simulink model "engineModelF16TestHarness"  (R2024a)
settings: configuration reference "standardSILConfiguraitonParams" (kept outside this file)
libraries: aerolibatmos2 x1
settings Model: Creator=jerem  LastModifiedBy=jerem
settings ConfigSetRef: SourceName=standardSILConfiguraitonParams  SourceLocation=Base Workspace

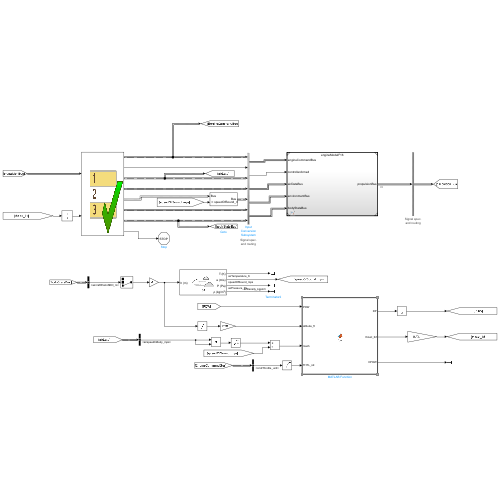
[thumbnail: Simulink's stored preview of the top-level diagram]
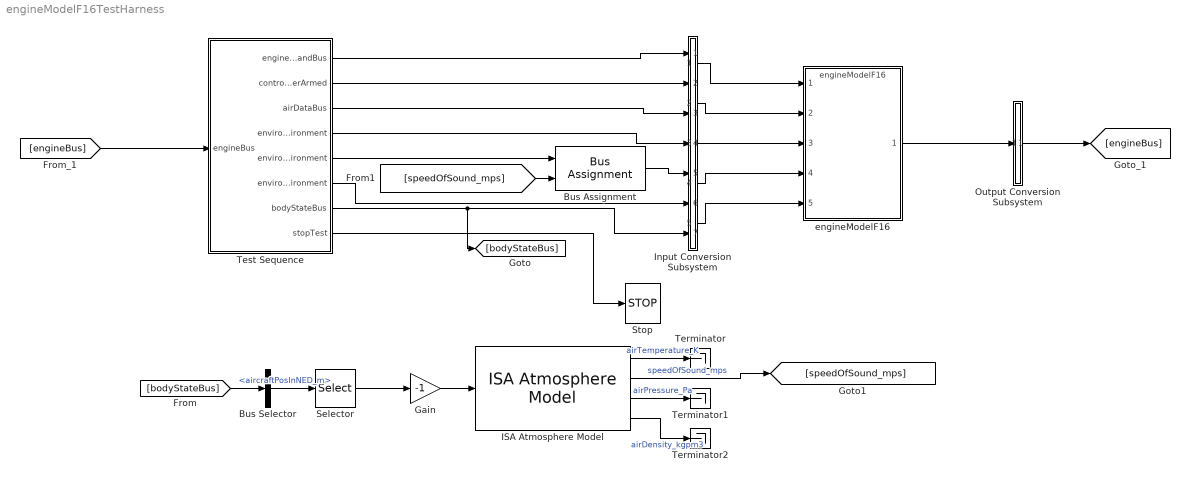
== system engineModelF16TestHarness ==
  Bus Assignment : BusAssignment  AssignedSignals=speedOfSound_mps
  Bus Selector : BusSelector  OutputSignals=aircraftPosInNED_m
  Gain : Gain  Gain=-1
  ISA Atmosphere Model : aerolibatmos2/ISA Atmosphere Model  useExtended=off  action=Warning  custom=off  viscosityOut=off  g=9.80665  gamma=1.4  R=287.0531  L=0.0065  h_trop=11000  h_strat=20000  rho0=1.225  P0=101325  T0=288.15  h0=0  S=110.4  Tref=273.15  muref=1.716e-5
  Input Conversion Subsystem : Subsystem  Tag=__SLT_ICS__  Description=|
      | Signal spec.
      | and routing
      settings: AttributesFormatString=%<Description>
  Output Conversion Subsystem : Subsystem  Tag=__SLT_OCS__  Description=|
      | Signal spec.
      | and routing
      mask init:
      | ICDictionary = get_param(bdroot, 'DataDictionary');
      | if isempty(ICDictionary)
      |    ICScope = Simulink.data.BaseWorkspace;
      | else
      |    ICScope = Simulink.data.DataDictionary(ICDictionary);
      | end
      | 
      | IC1 = Simulink.Bus.createMATLABStruct('EngineBus', [], [1 1], ICScope);
      settings: AttributesFormatString=%<Description>
  Selector : Selector  InputPortWidth=3  IndexOptions=Index vector (dialog)  Indices=3  OutputSizes=1
  Stop : Stop
  Terminator : Terminator
  Terminator1 : Terminator
  Terminator2 : Terminator
  Test Sequence : Test Sequence  TreatAsAtomicUnit=on
  engineModelF16 : ModelReference  ModelNameDialog=engineModelF16  SimulationMode=Normal  ModelReferenceVersion=1.84
  wires:
  Test Sequence/1(engineCommandBus) -> Input Conversion Subsystem/1(Inport_1)
  Test Sequence/2(controllerArmed) -> Input Conversion Subsystem/2(Inport_2)
  Test Sequence/3(airDataBus) -> Input Conversion Subsystem/3(Inport_3)
  Test Sequence/4(environmentBus_EarthEnvironment) -> Input Conversion Subsystem/4(Inport_4)
  Test Sequence/6(environmentBus_TerrainEnvironment) -> Input Conversion Subsystem/6(Inport_6)
  Test Sequence/7(bodyStateBus) -> [bodyStateBus], Input Conversion Subsystem/7(Inport_7)
  [engineBus] -> Test Sequence/1(engineBus)
  Output Conversion Subsystem/1(Outport_1) -> [engineBus]
  Input Conversion Subsystem/1(Outport_1) -> engineModelF16/1
  Input Conversion Subsystem/2(Outport_2) -> engineModelF16/2
  Input Conversion Subsystem/3(Outport_3) -> engineModelF16/3
  Input Conversion Subsystem/4(Outport_4) -> engineModelF16/4
  Input Conversion Subsystem/5(Outport_5) -> engineModelF16/5
  engineModelF16/1 -> Output Conversion Subsystem/1(Inport_1)
  Test Sequence/8(stopTest) -> Stop/1
  [bodyStateBus] -> Bus Selector/1
  Bus Selector/1 -> Selector/1  "<aircraftPosInNED_m>"
  Selector/1 -> Gain/1
  Gain/1 -> ISA Atmosphere Model/1
  ISA Atmosphere Model/1 -> Terminator/1  "airTemperature_K"
  ISA Atmosphere Model/3 -> Terminator1/1  "airPressure_Pa"
  ISA Atmosphere Model/4 -> Terminator2/1  "airDensity_kgpm3"
  ISA Atmosphere Model/2 -> [speedOfSound_mps]  "speedOfSound_mps"
  Test Sequence/5(environmentBus_AirEnvironment) -> Bus Assignment/1
  [speedOfSound_mps] -> Bus Assignment/2
  Bus Assignment/1 -> Input Conversion Subsystem/5(Inport_5)

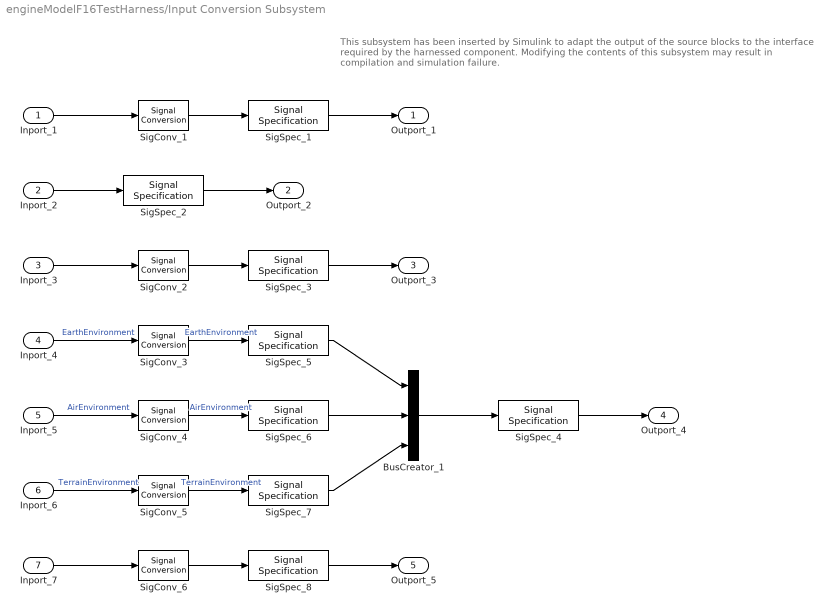
== system engineModelF16TestHarness/Input Conversion Subsystem ==
  note: This subsystem has been inserted by Simulink to adapt the output of the source blocks to the interface required by the harnessed component.
      |  Modifying the contents of this subsystem may result in compilation and simulation failure.
  Inport_1 : Inport
  Inport_2 : Inport  Port=2
  Inport_3 : Inport  Port=3
  Inport_4 : Inport  Port=4
  Inport_5 : Inport  Port=5
  Inport_6 : Inport  Port=6
  Inport_7 : Inport  Port=7
  BusCreator_1 : BusCreator  Inputs=3  OutDataTypeStr=Bus: EnvironmentBus
  SigConv_1 : SignalConversion  ConversionOutput=Virtual bus  OverrideOpt=off
  SigConv_2 : SignalConversion  ConversionOutput=Virtual bus  OverrideOpt=off
  SigConv_3 : SignalConversion  ConversionOutput=Nonvirtual bus  OverrideOpt=off
  SigConv_4 : SignalConversion  ConversionOutput=Nonvirtual bus  OverrideOpt=off
  SigConv_5 : SignalConversion  ConversionOutput=Nonvirtual bus  OverrideOpt=off
  SigConv_6 : SignalConversion  ConversionOutput=Virtual bus  OverrideOpt=off
  SigSpec_1 : SignalSpecification  OutDataTypeStr=Bus: EngineCommandBus  SampleTime=[-1, 0]
  SigSpec_2 : SignalSpecification  OutDataTypeStr=double  Dimensions=[1]  SampleTime=[-1, 0]
  SigSpec_3 : SignalSpecification  OutDataTypeStr=Bus: AirData  SampleTime=[-1, 0]
  SigSpec_4 : SignalSpecification  OutDataTypeStr=Bus: EnvironmentBus  SampleTime=[-1, 0]
  SigSpec_5 : SignalSpecification  OutDataTypeStr=Bus: EarthEnvironmentBus  Dimensions=[1]  SampleTime=[-1, 0]  BusOutputAsStruct=on
  SigSpec_6 : SignalSpecification  OutDataTypeStr=Bus: AirEnvironmentBus  Dimensions=[1]  SampleTime=[-1, 0]  BusOutputAsStruct=on
  SigSpec_7 : SignalSpecification  OutDataTypeStr=Bus: TerrainEnvironmentBus  Dimensions=[1]  SampleTime=[-1, 0]  BusOutputAsStruct=on
  SigSpec_8 : SignalSpecification  OutDataTypeStr=Bus: BodyStateBus  SampleTime=[-1, 0]
  Outport_1 : Outport
  Outport_2 : Outport  Port=2
  Outport_3 : Outport  Port=3
  Outport_4 : Outport  Port=4
  Outport_5 : Outport  Port=5
  wires:
  SigSpec_1/1 -> Outport_1/1
  SigConv_1/1 -> SigSpec_1/1
  Inport_1/1 -> SigConv_1/1
  SigSpec_2/1 -> Outport_2/1
  Inport_2/1 -> SigSpec_2/1
  SigSpec_3/1 -> Outport_3/1
  SigConv_2/1 -> SigSpec_3/1
  Inport_3/1 -> SigConv_2/1
  SigSpec_4/1 -> Outport_4/1
  BusCreator_1/1 -> SigSpec_4/1
  SigSpec_5/1 -> BusCreator_1/1
  SigConv_3/1 -> SigSpec_5/1  "EarthEnvironment"
  Inport_4/1 -> SigConv_3/1  "EarthEnvironment"
  SigSpec_6/1 -> BusCreator_1/2
  SigConv_4/1 -> SigSpec_6/1  "AirEnvironment"
  Inport_5/1 -> SigConv_4/1  "AirEnvironment"
  SigSpec_7/1 -> BusCreator_1/3
  SigConv_5/1 -> SigSpec_7/1  "TerrainEnvironment"
  Inport_6/1 -> SigConv_5/1  "TerrainEnvironment"
  SigSpec_8/1 -> Outport_5/1
  SigConv_6/1 -> SigSpec_8/1
  Inport_7/1 -> SigConv_6/1

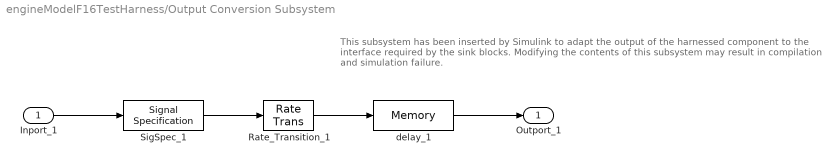
== system engineModelF16TestHarness/Output Conversion Subsystem ==
  note: This subsystem has been inserted by Simulink to adapt the output of the harnessed component to the interface required by the sink blocks.
      |  Modifying the contents of this subsystem may result in compilation and simulation failure.
  Inport_1 : Inport
  Rate_Transition_1 : RateTransition  OutPortSampleTimeOpt=Inherit
  SigSpec_1 : SignalSpecification  OutDataTypeStr=Bus: EngineBus  Dimensions=[1]
  delay_1 : Memory  InitialCondition=IC1
  Outport_1 : Outport
  wires:
  Inport_1/1 -> SigSpec_1/1
  SigSpec_1/1 -> Rate_Transition_1/1
  Rate_Transition_1/1 -> delay_1/1
  delay_1/1 -> Outport_1/1

== matlab function engineModelF16TestHarness/MATLAB Function ==
  data: POW input; DP output; altitude_ft input; mach input; thrust_lbf output; THTL_nd input; CPOW output
function [DP,thrust_lbf, CPOW] = fcn(POW, altitude_ft, mach, THTL_nd)

coder.extrinsic("PDOT")
coder.extrinsic("THRUST")
coder.extrinsic("TGEAR")
thrust_lbf = 0;
CPOW = 0;
DP = 0;

CPOW = TGEAR(THTL_nd);
thrust_lbf = THRUST(POW,altitude_ft, mach);
DP = PDOT(POW, CPOW);

== stateflow chart engineModelF16TestHarness/Test Sequence ==
  state Scenario_1
    state Initialize
      %% Initialize data outputs.
      engineCommandBus.cmdThrottle_unit = 0;
      controllerArmed = 0;
      airDataBus.airspeedInBody_mps = zeros(3,1);
      airDataBus.alpha_rad = 0;
      airDataBus.beta_rad = 0;
      environmentBus_EarthEnvironment.gravityScalar_mps2 = 0;
      environmentBus_EarthEnvironment.worldMagneticFieldInNED_nT = zeros(3,1);
      environmentBus_AirEnvironment.airTemperature_K = 0;
      environmentBus_AirEnvironment.airPressure_Pa = 0;
      environmentBus_AirEnvironment.airDensity_kgpm3 = 0;
      environmentBus_AirEnvironment.windSpeedInNED_mps = zeros(3,1);
      environmentBus_AirEnvironment.speedOfSound_mps = 0;
      environmentBus_AirEnvironment.windsAloftInNED_mps = zeros(3,1);
      environmentBus_AirEnvironment.gustInNED_mps = zeros(3,1);
      environmentBus_AirEnvironment.turbulenceInNED_mps = zeros(3,1);
      environmentBus_TerrainEnvironment.terrainHeightInNED_m = 0;
      bodyStateBus.aircraftVelInNED_mps = zeros(3,1);
      bodyStateBus.aircraftPosInNED_m = zeros(3,1);
      bodyStateBus.aircraftEulerAngles_rad = zeros(3,1);
      bodyStateBus.aircraftVelInBody_mps = zeros(3,1);
      bodyStateBus.aircraftAngVelInBody_radps = zeros(3,1);
      bodyStateBus.aircraftAngAccelInBody_radps2 = zeros(3,1);
      bodyStateBus.aircraftAccelInBody_mps2 = zeros(3,1);
      bodyStateBus.DCM_be = zeros(3,3);
      stopTest = false;
    state commandThrottle
      engineCommandBus.cmdThrottle_unit = 0.02;
    state verifyControllerDisarm
      verify(isClose(propulsionBus.engineForcesMoments.forcesInBody_N(1),0))
    state armController
      controllerArmed = 1;
      engineCommandBus.cmdThrottle_unit = 0.2;
    state verifyThorttle
      verify(isClose(thrust_lbf, propulsionBus.engineForcesMoments.forcesInBody_N(1), 'atol', 1))
    state maxCommandThrottle
      engineCommandBus.cmdThrottle_unit=10.5;
      settings: description=try out of range throttle > 1.0
    state verifyMaxThrust
      verify(propulsionBus.engineForcesMoments.forcesInBody_N(1) < 130000) % 130kN is what is listed on google as max thrust
      verify(isClose(thrust_lbf, propulsionBus.engineForcesMoments.forcesInBody_N(1), 'atol', 1))
      settings: description=max thrust taken from 5279e61a468c5ead544c0289877962cbf8e0459c
    state simulateAirspeed
      airDataBus.airspeedInBody_mps(1) = 100;
      bodyStateBus.aircraftPosInNED_m(3) = -1000;
    state verifyWithAirspeed
      verify(isClose(thrust_lbf, propulsionBus.engineForcesMoments.forcesInBody_N(1), 'atol', 1))
    state increaseAirspeed
      airDataBus.airspeedInBody_mps(1) = 250;
    state verifyIncreaseAirspeed
      verify(isClose(thrust_lbf, propulsionBus.engineForcesMoments.forcesInBody_N(1), 'atol', 1))
    state increaseAltitude
      bodyStateBus.aircraftPosInNED_m(3) = -12000;
    state verifyIncreaseAltitude
      verify(isClose(thrust_lbf, propulsionBus.engineForcesMoments.forcesInBody_N(1), 'atol', 1))
    state EndTest
      stopTest = true;
    (default) -> Initialize
    Initialize -> commandThrottle : [
        | true
        | ]
    commandThrottle -> verifyControllerDisarm : [
        | after(2,sec)
        | ]
    verifyControllerDisarm -> armController : [
        | after(1,sec)
        | ]
    armController -> verifyThorttle : [
        | after(6,sec)
        | ]
    verifyThorttle -> maxCommandThrottle : [
        | after(1,sec)
        | ]
    maxCommandThrottle -> verifyMaxThrust : [
        | after(6,sec)
        | ]
    verifyMaxThrust -> simulateAirspeed : [
        | after(1, sec)
        | ]
    simulateAirspeed -> verifyWithAirspeed : [
        | after(6,sec)
        | ]
    verifyWithAirspeed -> increaseAirspeed : [
        | after(1,sec)
        | ]
    increaseAirspeed -> verifyIncreaseAirspeed : [
        | after(6,sec)
        | ]
    verifyIncreaseAirspeed -> increaseAltitude : [
        | after(1,sec)
        | ]
    increaseAltitude -> verifyIncreaseAltitude : [
        | after(6,sec)
        | ]
    verifyIncreaseAltitude -> EndTest : [
        | after(1,sec)
        | ]
  (default) -> Scenario_1 : {assert(Active_Scenario_Index == 1,'The value of Scenario Parameter ''Active_Scenario_Index'' is not valid. Use the index of the scenario to specify it.')}
  data: propulsionBus input Bus: PropulsionBus size=[1]; engineCommandBus output Bus: EngineCommandBus size=[1]; controllerArmed output double size=[1]; airDataBus output Bus: AirDataBus size=[1]; environmentBus_EarthEnvironment output Bus: EarthEnvironmentBus size=[1]; environmentBus_AirEnvironment output Bus: AirEnvironmentBus size=[1]; environmentBus_TerrainEnvironment output Bus: TerrainEnvironmentBus size=[1]; bodyStateBus output Bus: BodyStateBus size=[1]; stopTest output; Active_Scenario_Index parameter =1; thrust_lbf input
